simulink model "DKTN_MRAC_MIENROIRAC"  (R2023a)
settings: Solver=FixedStepDiscrete  StartTime=0.0  StopTime=100  FixedStep=0.005  RelTol=1e-3
undefined symbols (not defined in the file or in its folder): DiscIntNeverNeededParam
libraries: simulink x1, SignalEditorBlockLib x1
settings Model: Creator=FPTSHOP  LastModifiedBy=FPTSHOP

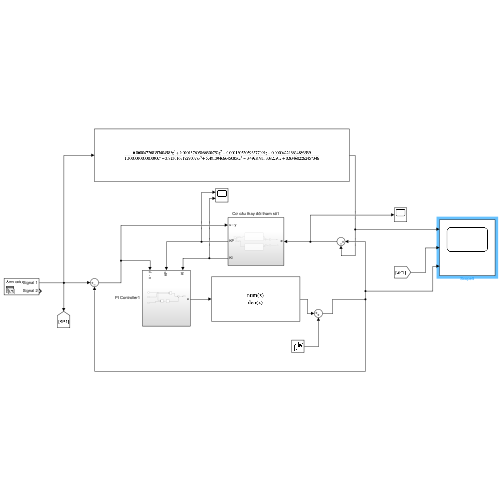
[thumbnail: Simulink's stored preview of the top-level diagram]
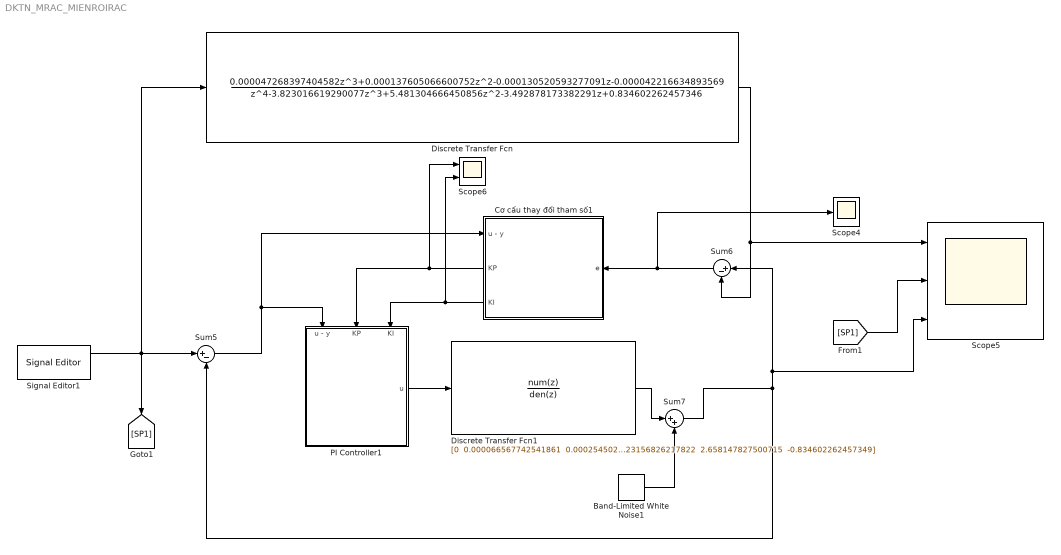
== system DKTN_MRAC_MIENROIRAC ==
  Band-Limited White Noise1 : simulink/Sources/Band-Limited White Noise  Cov=[0.0001]  Ts=0.1  seed=[23341]
  Cơ cấu thay đổi tham số1 : Subsystem
      settings: PortSchema="{\"entries\":[{\"content\":{\"sides\":[{\"content\":{\"connectorIds\":[\"In1\"]},\"type\":\"ConnectorPlacement.EquallySpacedRectSide\",\"uuid\":\"80899429-ec5e-4ea6-9130-530fe1f37aef\"},{\"content\":{\"connectorIds\":[\"In2\",\"Out1\",\"Out2\"],\"side\":\"RIGHT\"},\"type\":\"ConnectorPlacement.EquallySpacedRectSide\",\"uuid\":\"4a2de49c-21b3-4ae3-b9e0-d77aef8f9de0\"},{\"content\":{\"side\":\"TOP\"},\"type\":\"ConnectorPlacement.EquallySpacedRectSide\",\"uuid\":\"a7b60cec-568b-41d4-926d-6ff42a0e1872\"},{\"content\":{\"side\":\"BOTTOM\"},\"type\":\"ConnectorPlacement.EquallySpacedRectSide\",\"uuid\":\"44227394-6553-42ce-9b91-3aff6074a502\"}]},\"type\":\"ConnectorPlacement.EquallySpacedConnector\",\"uuid\":\"655fcbc3-75b2-4ba4-9e50-e4789fbe396c\"}],\"packageUris\":[\"http://schema.mathworks.com/mf0/Connector/R2020b\"],\"version\":\"1.0\"}"
  Discrete Transfer Fcn : DiscreteTransferFcn  Numerator="[0  0.000047268397404582  0.000137605066600752  -0.000130520593277091  -0.000042216634893569]"  Denominator="[1.000000000000000  -3.823016619290077   5.481304666450856  -3.492878173382291   0.834602262457346]"  SampleTime=0.005
  Discrete Transfer Fcn1 : DiscreteTransferFcn  Numerator="[0  0.000066567742541861  0.000254502975927928  0.000060814057842816]"  Denominator="[1.000000000000000  -2.823156826217822  2.658147827500715  -0.834602262457349]"  SampleTime=0.005
  PI Controller1 : Subsystem
      settings: PortSchema="{\"entries\":[{\"content\":{\"sides\":[{\"content\":{\"connectorIds\":[\"In1\",\"In2\",\"In3\"]},\"type\":\"ConnectorPlacement.EquallySpacedRectSide\",\"uuid\":\"dddaaed2-e507-451a-921f-c04901101d86\"},{\"content\":{\"side\":\"RIGHT\"},\"type\":\"ConnectorPlacement.EquallySpacedRectSide\",\"uuid\":\"ae8720e4-d060-4dea-b1b4-5825fbf776f2\"},{\"content\":{\"side\":\"TOP\"},\"type\":\"ConnectorPlacement.EquallySpacedRectSide\",\"uuid\":\"05c90be4-7f2e-46e3-b0ab-720f61a4a343\"},{\"content\":{\"connectorIds\":[\"Out1\"],\"side\":\"BOTTOM\"},\"type\":\"ConnectorPlacement.EquallySpacedRectSide\",\"uuid\":\"f7a2217c-f25e-4afe-a869-2b8c8d87a3a7\"}]},\"type\":\"ConnectorPlacement.EquallySpacedConnector\",\"uuid\":\"e4383ad1-63b6-41a4-973a-f7aa36cab285\"}],\"packageUris\":[\"http://schema.mathworks.com/mf0/Connector/R2020b\"],\"version\":\"1.0\"}"
  Scope4 : Scope
  Scope5 : Scope  NumInputPorts=3
  Scope6 : Scope  NumInputPorts=2
  Signal Editor1 : SignalEditorBlockLib/Signal Editor  FileName=I:\DUT\DK Thich Nghi\CUOIKI\signal.mat  ActiveScenario=Scenario  ActiveSignal=Signal 1  IsBus=off  OutputBusObjectStr=Bus: BusObject  SampleTime=0  Interpolate=off  ZeroCross=off  OutputAfterFinalValue=Setting to zero  Unit=inherit  PreserveSignalName=on  ApplySigPropsToAllScenarios=on
  Sum5 : Sum  Inputs=|+-
  Sum6 : Sum  Inputs=|+-
  Sum7 : Sum  Inputs=|++
  wires:
  Sum6/1 -> Scope4/1, Cơ cấu thay đổi tham số1/1(e)
  Sum7/1 -> Scope5/3, Sum6/1, Sum5/2
  Discrete Transfer Fcn1/1 -> Sum7/1
  Cơ cấu thay đổi tham số1/1(KP) -> Scope6/1, PI Controller1/2(KP)
  Cơ cấu thay đổi tham số1/2(KI) -> Scope6/2, PI Controller1/3(KI)
  Sum5/1 -> PI Controller1/1(u - y), Cơ cấu thay đổi tham số1/2(u - y)
  Signal Editor1/1 -> Discrete Transfer Fcn/1, [SP1], Sum5/1
  [SP1] -> Scope5/2
  Discrete Transfer Fcn/1 -> Scope5/1, Sum6/2
  PI Controller1/1(u) -> Discrete Transfer Fcn1/1
  Band-Limited White Noise1/1 -> Sum7/2

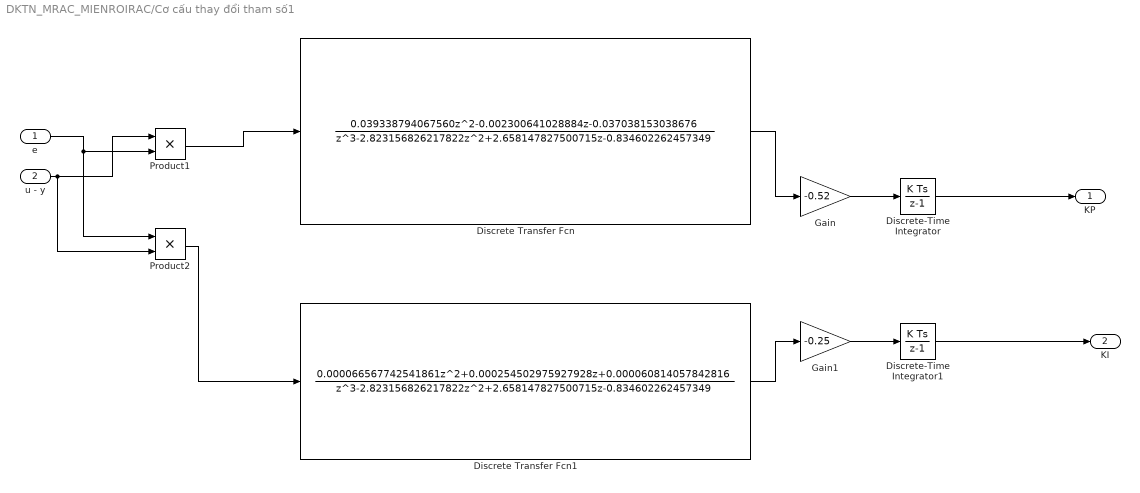
== system DKTN_MRAC_MIENROIRAC/Cơ cấu thay đổi tham số1 ==
  e : Inport
  u - y : Inport  Port=2
  Discrete Transfer Fcn : DiscreteTransferFcn  Numerator="[0   0.039338794067560  -0.002300641028884  -0.037038153038676]"  Denominator="[1.000000000000000  -2.823156826217822   2.658147827500715  -0.834602262457349]"  SampleTime=0.005
  Discrete Transfer Fcn1 : DiscreteTransferFcn  Numerator="[0  0.000066567742541861  0.000254502975927928  0.000060814057842816]"  Denominator="[1.000000000000000  -2.823156826217822   2.658147827500715  -0.834602262457349]"  SampleTime=0.005
  Discrete-Time Integrator : DiscreteIntegrator  SampleTime=0.005  ICPrevOutput=DiscIntNeverNeededParam  ICPrevScaledInput=DiscIntNeverNeededParam
  Discrete-Time Integrator1 : DiscreteIntegrator  SampleTime=0.005  ICPrevOutput=DiscIntNeverNeededParam  ICPrevScaledInput=DiscIntNeverNeededParam
  Gain : Gain  Gain=-0.52
  Gain1 : Gain  Gain=-0.25
  Product1 : Product
  Product2 : Product
  KP : Outport
  KI : Outport  Port=2
  wires:
  Discrete Transfer Fcn/1 -> Gain/1
  Gain/1 -> Discrete-Time Integrator/1
  Discrete Transfer Fcn1/1 -> Gain1/1
  Gain1/1 -> Discrete-Time Integrator1/1
  e/1 -> Product2/1, Product1/2
  u - y/1 -> Product2/2, Product1/1
  Product1/1 -> Discrete Transfer Fcn/1
  Product2/1 -> Discrete Transfer Fcn1/1
  Discrete-Time Integrator/1 -> KP/1
  Discrete-Time Integrator1/1 -> KI/1

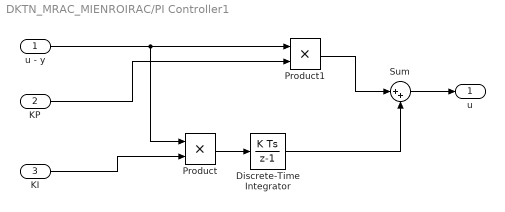
== system DKTN_MRAC_MIENROIRAC/PI Controller1 ==
  u - y : Inport
  KP : Inport  Port=2
  KI : Inport  Port=3
  Discrete-Time Integrator : DiscreteIntegrator  SampleTime=0.005  ICPrevOutput=DiscIntNeverNeededParam  ICPrevScaledInput=DiscIntNeverNeededParam
  Product : Product
  Product1 : Product
  Sum : Sum  Inputs=|++
  u : Outport
  wires:
  KP/1 -> Product1/2
  u - y/1 -> Product/1, Product1/1
  Sum/1 -> u/1
  Product1/1 -> Sum/1
  KI/1 -> Product/2
  Product/1 -> Discrete-Time Integrator/1
  Discrete-Time Integrator/1 -> Sum/2
